simulink model "Buck_closed_loop_analog_control"  (R2019a)
settings: Solver=ode45  StartTime=0.0  StopTime=0.03  MaxStep=0.1e-6  RelTol=1e-3  EnableMultiTasking=on
libraries: simulink x4
settings Model: Creator=Rony  LastModifiedBy=asus
settings DataIOCC: LimitDataPoints=on  SaveFormat=Array  ReturnWorkspaceOutputs=off
settings OptimizationCC: LifeSpan=inf
settings DebuggingCC: UnderspecifiedInitializationDetection=Classic  MergeDetectMultiDrivingBlocksExec=none  SolverPrmCheckMsg=warning  StateNameClashWarn=warning  SFUnexpectedBacktrackingDiag=warning  SFNoUnconditionalDefaultTransitionDiag=warning  SFExecutionAtInitializationDiag=none  ArithmeticOperatorsInVariantConditions=warning
settings HardwareCC: ProdBitPerPointer=32  ProdBitPerSizeT=32  ProdBitPerPtrDiffT=32  ProdLargestAtomicFloat=None  ProdIntDivRoundTo=Undefined  ProdEndianess=Unspecified  ProdWordSize=32  ProdHWDeviceType=32-bit Generic
settings ModelReferenceCC: PropagateSignalLabelsOutOfModel=off
settings SFSimCC: SimUseLocalCustomCode=off
settings RTWCC: RTWUseLocalCustomCode=off
settings CodeAppCC: StateflowObjectComments=on
settings GRTTargetCC: TargetLangStandard=C89/C90 (ANSI)  GeneratePreprocessorConditionals=Disable all
settings ConfigComp: CovMetricSettings=dw  CovHtmlReporting=on  CovSaveCumulativeToWorkspaceVar=on  CovSaveSingleToWorkspaceVar=on  CovExternalEMLEnable=off

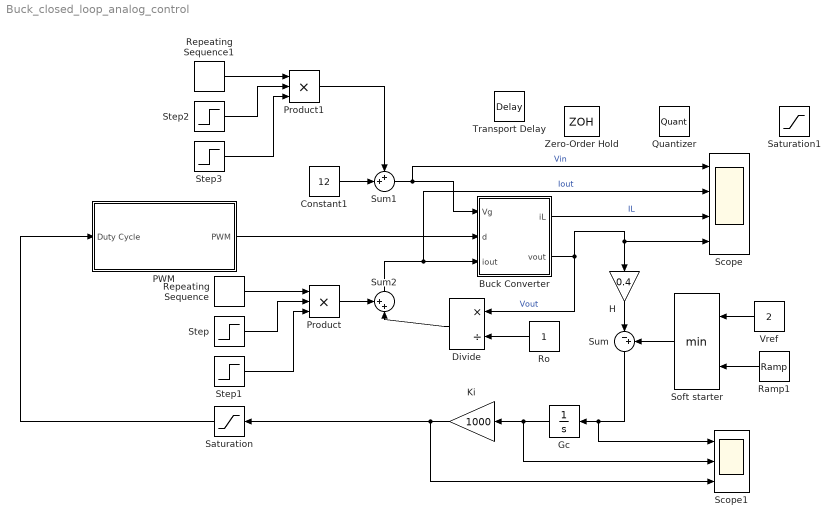
== system Buck_closed_loop_analog_control ==
  Buck Converter : Subsystem
  Constant1 : Constant  Value=12
  Divide : Product  Inputs=*/
  Gc : Integrator  UpperSaturationLimit=0.9/1000  LowerSaturationLimit=0.1/1000
  H : Gain  Gain=0.4
  Ki : Gain  Gain=1000
  PWM : Subsystem
  Product : Product  Inputs=3
  Product1 : Product  Inputs=3
  Quantizer : Quantizer  QuantizationInterval=1/64
  Ramp1 : simulink/Sources/Ramp  slope=2/(25e-6)  start=0  InitialOutput=0
  Repeating Sequence : simulink/Sources/Repeating Sequence  rep_seq_t="[0 1000e-6  1001e-6 1002e-6 2000e-6 2001e-6 2002e-6]"  rep_seq_y="[-5  -5  0 5 5 0 -5]"
  Repeating Sequence1 : simulink/Sources/Repeating Sequence  rep_seq_t="[0 2000e-6  2001e-6 2002e-6 4000e-6 4001e-6 4002e-6]"  rep_seq_y="[-5  -5  0 5 5 0 -5]"
  Ro : Constant
  Saturation : Saturate  UpperLimit=0.9  LowerLimit=0.05
  Saturation1 : Saturate  UpperLimit=1  LowerLimit=-1
  Scope : Scope  NumInputPorts=4
  Scope1 : Scope  NumInputPorts=3
  "Soft starter " : MinMax  Inputs=2
  Step : Step  Time=.01  SampleTime=0
  Step1 : Step  Time=.013  Before=1  After=0  SampleTime=0
  Step2 : Step  Time=.02  SampleTime=0
  Step3 : Step  Time=.023  Before=1  After=0  SampleTime=0
  Sum : Sum  Inputs=|-+
  Sum1 : Sum  Inputs=++|
  Sum2 : Sum  Inputs=++|
  Transport Delay : TransportDelay  DelayTime=4e-6
  Vref : Constant  Value=2
  Zero-Order Hold : ZeroOrderHold  SampleTime=10e-6
  wires:
  Buck Converter/1(iL) -> Scope/3  "IL"
  Buck Converter/2("vout ") -> H/1, Scope/4, Divide/1  "Vout"
  Ki/1 -> Scope1/3, Saturation/1
  PWM/1(PWM) -> Buck Converter/2(d)
  H/1 -> Sum/1
  Gc/1 -> Scope1/2, Ki/1
  Ro/1 -> Divide/2
  Constant1/1 -> Sum1/2
  Sum1/1 -> Scope/1, Buck Converter/1(Vg)  "Vin"
  Saturation/1 -> PWM/1(Duty Cycle)
  Divide/1 -> Sum2/2
  Sum2/1 -> Scope/2, Buck Converter/3(iout)  "Iout"
  Repeating Sequence/1 -> Product/1
  Step/1 -> Product/2
  Product/1 -> Sum2/1
  "Soft starter "/1 -> Sum/2
  Ramp1/1 -> "Soft starter "/2
  Vref/1 -> "Soft starter "/1
  Sum/1 -> Scope1/1, Gc/1
  Step1/1 -> Product/3
  Step3/1 -> Product1/3
  Product1/1 -> Sum1/1
  Step2/1 -> Product1/2
  Repeating Sequence1/1 -> Product1/1

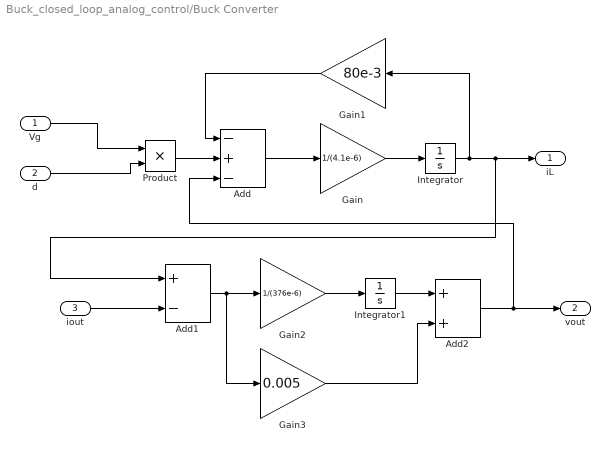
== system Buck_closed_loop_analog_control/Buck Converter ==
  Vg : Inport
  d : Inport  Port=2
  iout : Inport  Port=3
  Add : Sum  Inputs=-+-
  Add1 : Sum  Inputs=+-
  Add2 : Sum
  Gain : Gain  Gain=1/(4.1e-6)
  Gain1 : Gain  Gain=80e-3
  Gain2 : Gain  Gain=1/(376e-6)
  Gain3 : Gain  Gain=0.005
  Integrator : Integrator
  Integrator1 : Integrator
  Product : Product
  iL : Outport
  "vout " : Outport  Port=2
  wires:
  Add/1 -> Gain/1
  Vg/1 -> Product/1
  d/1 -> Product/2
  Add2/1 -> "vout "/1, Add/3
  Gain/1 -> Integrator/1
  Integrator/1 -> iL/1, Add1/1, Gain1/1
  Product/1 -> Add/2
  Integrator1/1 -> Add2/1
  Add1/1 -> Gain3/1, Gain2/1
  Gain3/1 -> Add2/2
  Gain1/1 -> Add/1
  iout/1 -> Add1/2
  Gain2/1 -> Integrator1/1

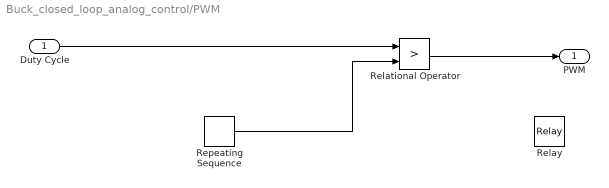
== system Buck_closed_loop_analog_control/PWM ==
  Duty Cycle : Inport
  Relational Operator : RelationalOperator  Operator=>  OutDataTypeStr=boolean  RndMeth=Nearest
  Relay : Relay
  Repeating Sequence : simulink/Sources/Repeating Sequence  rep_seq_t=[0 0.001e-5 1e-5]  rep_seq_y=[1 0 1]
  PWM : Outport
  wires:
  Relational Operator/1 -> PWM/1
  Repeating Sequence/1 -> Relational Operator/2
  Duty Cycle/1 -> Relational Operator/1
